simulink model "TorqueDistribution"  (R2024b)
settings: configuration reference "STM32H7_Config" (kept outside this file)
undefined symbols (not defined in the file): MMotorMaxAllowed, MMotorMinAllowed, MNominal, NKe
libraries: simulink x5
settings Model: DataDictionary=Master_Dictionary.sldd  EnableAccessToBaseWorkspace=off  Creator=torni  LastModifiedBy=William
settings ConfigSetRef: SourceName=STM32H7_Config

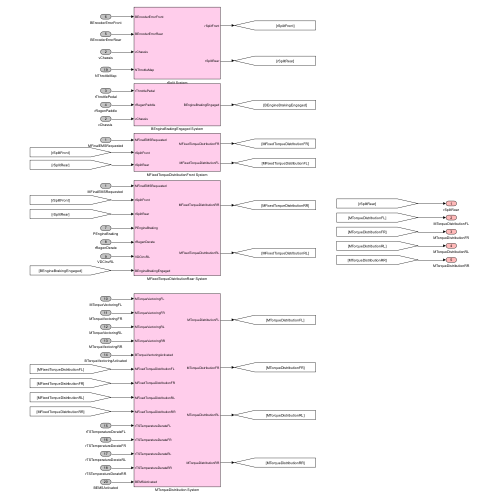
[thumbnail: Simulink's stored preview of the top-level diagram]
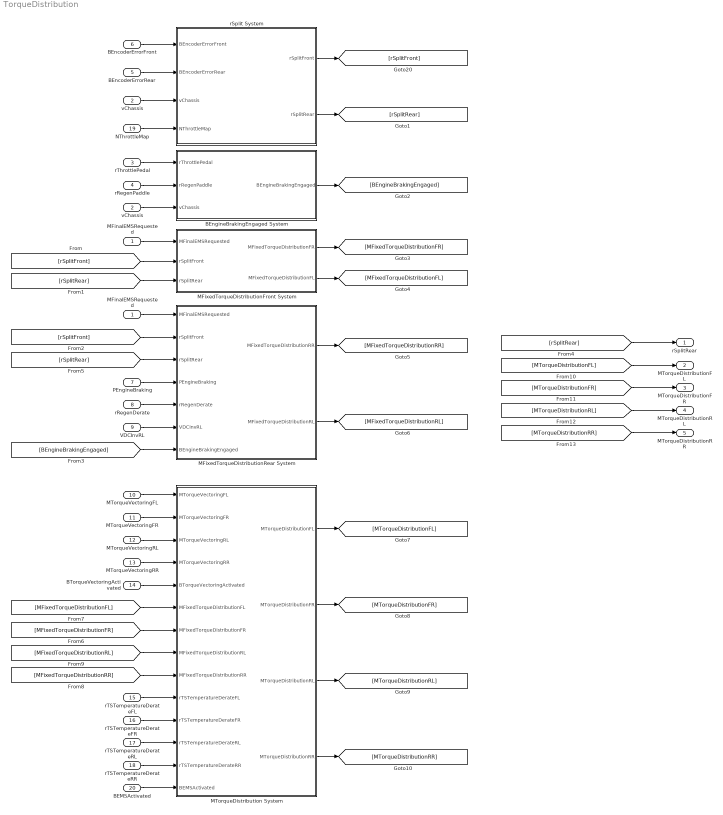
== system TorqueDistribution ==
  MFinalEMSRequested : Inport  OutDataTypeStr=double
  vChassis : Inport  Port=2  OutDataTypeStr=double
  "rThrottlePedal " : Inport  Port=3  OutDataTypeStr=double
  rRegenPaddle : Inport  Port=4  OutDataTypeStr=double
  BEncoderErrorRear : Inport  Port=5  OutDataTypeStr=boolean
  BEncoderErrorFront : Inport  Port=6  OutDataTypeStr=boolean
  PEngineBraking : Inport  Port=7  OutDataTypeStr=double
  rRegenDerate : Inport  Port=8  OutDataTypeStr=double
  VDCInvRL : Inport  Port=9  OutDataTypeStr=double
  MTorqueVectoringFL : Inport  Port=10  OutDataTypeStr=double
  MTorqueVectoringFR : Inport  Port=11  OutDataTypeStr=double
  MTorqueVectoringRL : Inport  Port=12  OutDataTypeStr=double
  MTorqueVectoringRR : Inport  Port=13  OutDataTypeStr=double
  BTorqueVectoringActivated : Inport  Port=14  OutDataTypeStr=boolean
  rTSTemperatureDerateFL : Inport  Port=15  OutDataTypeStr=double
  rTSTemperatureDerateFR : Inport  Port=16  OutDataTypeStr=double
  rTSTemperatureDerateRL : Inport  Port=17  OutDataTypeStr=double
  rTSTemperatureDerateRR : Inport  Port=18  OutDataTypeStr=double
  NThrottleMap : Inport  Port=19  OutDataTypeStr=double
  BEMSActivated : Inport  Port=20  OutDataTypeStr=boolean
  BEngineBrakingEngaged System : Subsystem
  "MFinalEMSRequested " : InportShadow  OutDataTypeStr=double
  MFixedTorqueDistributionFront System : Subsystem
  MFixedTorqueDistributionRear System : Subsystem
  MTorqueDistribution System : Subsystem
  rSplit System : Subsystem
  "vChassis " : InportShadow  Port=2  OutDataTypeStr=double
  rSplitRear : Outport  OutDataTypeStr=double  VectorParamsAs1DForOutWhenUnconnected=off
  MTorqueDistributionFL : Outport  Port=2  OutDataTypeStr=double  VectorParamsAs1DForOutWhenUnconnected=off
  MTorqueDistributionFR : Outport  Port=3  OutDataTypeStr=double  VectorParamsAs1DForOutWhenUnconnected=off
  MTorqueDistributionRL : Outport  Port=4  OutDataTypeStr=double  VectorParamsAs1DForOutWhenUnconnected=off
  MTorqueDistributionRR : Outport  Port=5  OutDataTypeStr=double  VectorParamsAs1DForOutWhenUnconnected=off
  wires:
  MFinalEMSRequested/1 -> MFixedTorqueDistributionFront System/1(MFinalEMSRequested)
  [rSplitRear] -> rSplitRear/1
  vChassis/1 -> rSplit System/3(vChassis)
  BEncoderErrorRear/1 -> rSplit System/2(BEncoderErrorRear)
  BEncoderErrorFront/1 -> rSplit System/1(BEncoderErrorFront)
  rSplit System/1(rSplitFront) -> [rSplitFront]
  rSplit System/2(rSplitRear) -> [rSplitRear]
  [rSplitFront] -> MFixedTorqueDistributionFront System/2(rSplitFront)
  [rSplitRear] -> MFixedTorqueDistributionFront System/3(rSplitRear)
  "rThrottlePedal "/1 -> BEngineBrakingEngaged System/1("rThrottlePedal ")
  rRegenPaddle/1 -> BEngineBrakingEngaged System/2(rRegenPaddle)
  BEngineBrakingEngaged System/1(BEngineBrakingEngaged) -> [BEngineBrakingEngaged]
  "MFinalEMSRequested "/1 -> MFixedTorqueDistributionRear System/1(MFinalEMSRequested)
  [rSplitFront] -> MFixedTorqueDistributionRear System/2(rSplitFront)
  [BEngineBrakingEngaged] -> MFixedTorqueDistributionRear System/7(BEngineBrakingEngaged)
  [rSplitRear] -> MFixedTorqueDistributionRear System/3(rSplitRear)
  PEngineBraking/1 -> MFixedTorqueDistributionRear System/4(PEngineBraking)
  rRegenDerate/1 -> MFixedTorqueDistributionRear System/5(rRegenDerate)
  VDCInvRL/1 -> MFixedTorqueDistributionRear System/6(VDCInvRL)
  MFixedTorqueDistributionFront System/1(MFixedTorqueDistributionFR) -> [MFixedTorqueDistributionFR]
  MFixedTorqueDistributionFront System/2(MFixedTorqueDistributionFL) -> [MFixedTorqueDistributionFL]
  MFixedTorqueDistributionRear System/1(MFixedTorqueDistributionRR) -> [MFixedTorqueDistributionRR]
  MFixedTorqueDistributionRear System/2(MFixedTorqueDistributionRL) -> [MFixedTorqueDistributionRL]
  [MFixedTorqueDistributionFL] -> MTorqueDistribution System/6("MFixedTorqueDistributionFL ")
  [MFixedTorqueDistributionFR] -> MTorqueDistribution System/7(MFixedTorqueDistributionFR)
  [MFixedTorqueDistributionRL] -> MTorqueDistribution System/8(MFixedTorqueDistributionRL)
  [MFixedTorqueDistributionRR] -> MTorqueDistribution System/9(MFixedTorqueDistributionRR)
  MTorqueVectoringFL/1 -> MTorqueDistribution System/1(MTorqueVectoringFL)
  MTorqueVectoringFR/1 -> MTorqueDistribution System/2(MTorqueVectoringFR)
  MTorqueVectoringRL/1 -> MTorqueDistribution System/3(MTorqueVectoringRL)
  MTorqueVectoringRR/1 -> MTorqueDistribution System/4(MTorqueVectoringRR)
  BTorqueVectoringActivated/1 -> MTorqueDistribution System/5(BTorqueVectoringActivated)
  MTorqueDistribution System/1(MTorqueDistributionFL) -> [MTorqueDistributionFL]
  MTorqueDistribution System/2(MTorqueDistributionFR) -> [MTorqueDistributionFR]
  MTorqueDistribution System/3(MTorqueDistributionRL) -> [MTorqueDistributionRL]
  MTorqueDistribution System/4(MTorqueDistributionRR) -> [MTorqueDistributionRR]
  [MTorqueDistributionFL] -> MTorqueDistributionFL/1
  [MTorqueDistributionFR] -> MTorqueDistributionFR/1
  [MTorqueDistributionRL] -> MTorqueDistributionRL/1
  [MTorqueDistributionRR] -> MTorqueDistributionRR/1
  rTSTemperatureDerateFL/1 -> MTorqueDistribution System/10(rTSTemperatureDerateFL)
  rTSTemperatureDerateFR/1 -> MTorqueDistribution System/11(rTSTemperatureDerateFR)
  rTSTemperatureDerateRL/1 -> MTorqueDistribution System/12(rTSTemperatureDerateRL)
  rTSTemperatureDerateRR/1 -> MTorqueDistribution System/13(rTSTemperatureDerateRR)
  "vChassis "/1 -> BEngineBrakingEngaged System/3(vChassis)
  NThrottleMap/1 -> rSplit System/4(NThrottleMap)
  BEMSActivated/1 -> MTorqueDistribution System/14(BEMSActivated)

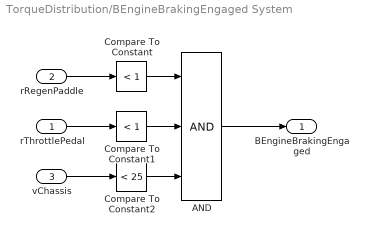
== system TorqueDistribution/BEngineBrakingEngaged System ==
  "rThrottlePedal " : Inport  OutDataTypeStr=double
  rRegenPaddle : Inport  Port=2  OutDataTypeStr=double
  vChassis : Inport  Port=3  OutDataTypeStr=double
  AND : Logic  Inputs=3  AllPortsSameDT=off  OutDataTypeStr=boolean
  Compare To Constant : simulink/Logic and Bit Operations/Compare To Constant  relop=<  const=1  OutDataTypeStr=boolean
  Compare To Constant1 : simulink/Logic and Bit Operations/Compare To Constant  relop=<  const=1  OutDataTypeStr=boolean
  Compare To Constant2 : simulink/Logic and Bit Operations/Compare To Constant  relop=<  const=25  OutDataTypeStr=boolean
  BEngineBrakingEngaged : Outport  OutDataTypeStr=boolean  VectorParamsAs1DForOutWhenUnconnected=off
  wires:
  AND/1 -> BEngineBrakingEngaged/1
  rRegenPaddle/1 -> Compare To Constant/1
  Compare To Constant1/1 -> AND/2
  Compare To Constant/1 -> AND/1
  "rThrottlePedal "/1 -> Compare To Constant1/1
  vChassis/1 -> Compare To Constant2/1
  Compare To Constant2/1 -> AND/3

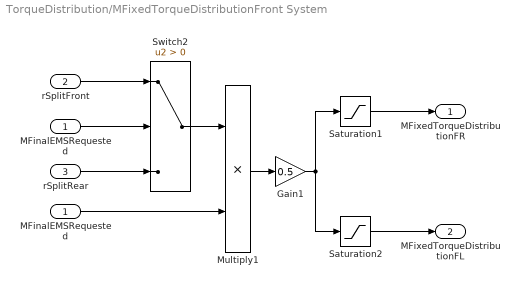
== system TorqueDistribution/MFixedTorqueDistributionFront System ==
  MFinalEMSRequested : Inport  OutDataTypeStr=double
  rSplitFront : Inport  Port=2  OutDataTypeStr=double
  rSplitRear : Inport  Port=3  OutDataTypeStr=double
  Gain1 : Gain  Gain=0.5
  "MFinalEMSRequested " : InportShadow  OutDataTypeStr=double
  Multiply1 : Product
  Saturation1 : Saturate  UpperLimit=MMotorMaxAllowed  LowerLimit=MMotorMinAllowed
  Saturation2 : Saturate  UpperLimit=MMotorMaxAllowed  LowerLimit=MMotorMinAllowed
  Switch2 : Switch  Criteria=u2 > Threshold  SaturateOnIntegerOverflow=off  InputSameDT=off
  MFixedTorqueDistributionFR : Outport  OutDataTypeStr=double  VectorParamsAs1DForOutWhenUnconnected=off
  MFixedTorqueDistributionFL : Outport  Port=2  OutDataTypeStr=double  VectorParamsAs1DForOutWhenUnconnected=off
  wires:
  Saturation2/1 -> MFixedTorqueDistributionFL/1
  Switch2/1 -> Multiply1/1
  Saturation1/1 -> MFixedTorqueDistributionFR/1
  Gain1/1 -> Saturation2/1, Saturation1/1
  Multiply1/1 -> Gain1/1
  MFinalEMSRequested/1 -> Switch2/2
  rSplitFront/1 -> Switch2/1
  rSplitRear/1 -> Switch2/3
  "MFinalEMSRequested "/1 -> Multiply1/2

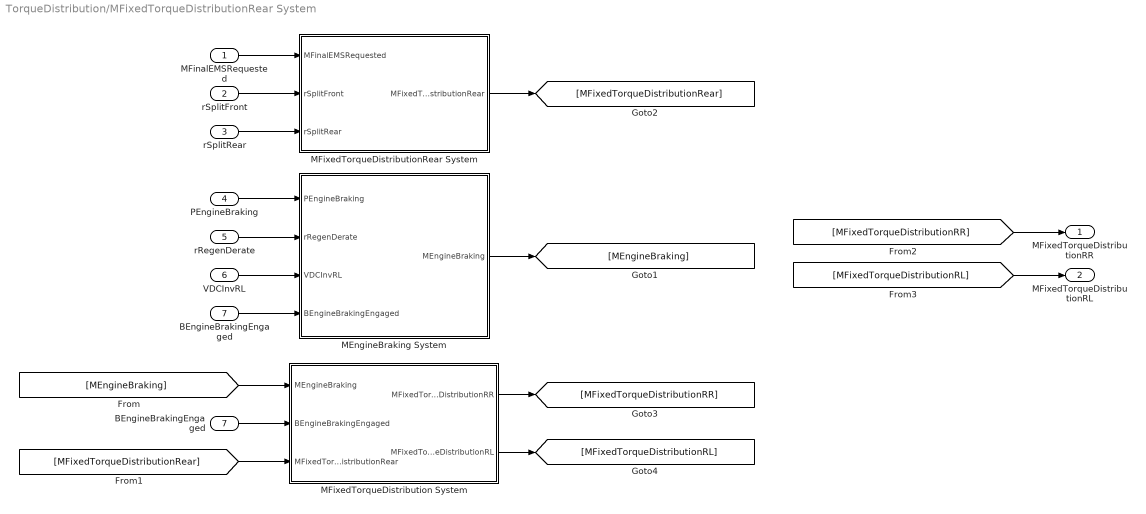
== system TorqueDistribution/MFixedTorqueDistributionRear System ==
  MFinalEMSRequested : Inport  OutDataTypeStr=double
  rSplitFront : Inport  Port=2  OutDataTypeStr=double
  rSplitRear : Inport  Port=3  OutDataTypeStr=double
  PEngineBraking : Inport  Port=4  OutDataTypeStr=double
  rRegenDerate : Inport  Port=5  OutDataTypeStr=double
  VDCInvRL : Inport  Port=6  OutDataTypeStr=double
  BEngineBrakingEngaged : Inport  Port=7  OutDataTypeStr=boolean
  "BEngineBrakingEngaged " : InportShadow  Port=7  OutDataTypeStr=boolean
  MEngineBraking System : Subsystem
  MFixedTorqueDistribution System : Subsystem
  MFixedTorqueDistributionRear System : Subsystem
  MFixedTorqueDistributionRR : Outport  OutDataTypeStr=double  VectorParamsAs1DForOutWhenUnconnected=off
  MFixedTorqueDistributionRL : Outport  Port=2  OutDataTypeStr=double  VectorParamsAs1DForOutWhenUnconnected=off
  wires:
  MFinalEMSRequested/1 -> MFixedTorqueDistributionRear System/1(MFinalEMSRequested)
  rSplitFront/1 -> MFixedTorqueDistributionRear System/2(rSplitFront)
  rSplitRear/1 -> MFixedTorqueDistributionRear System/3(rSplitRear)
  MFixedTorqueDistributionRear System/1(MFixedTorqueDistributionRear) -> [MFixedTorqueDistributionRear]
  PEngineBraking/1 -> MEngineBraking System/1(PEngineBraking)
  rRegenDerate/1 -> MEngineBraking System/2(rRegenDerate)
  VDCInvRL/1 -> MEngineBraking System/3(VDCInvRL)
  BEngineBrakingEngaged/1 -> MEngineBraking System/4(BEngineBrakingEngaged)
  MEngineBraking System/1(MEngineBraking) -> [MEngineBraking]
  "BEngineBrakingEngaged "/1 -> MFixedTorqueDistribution System/2(BEngineBrakingEngaged)
  [MEngineBraking] -> MFixedTorqueDistribution System/1(MEngineBraking)
  [MFixedTorqueDistributionRear] -> MFixedTorqueDistribution System/3(MFixedTorqueDistributionRear)
  MFixedTorqueDistribution System/1(MFixedTorqueDistributionRR) -> [MFixedTorqueDistributionRR]
  MFixedTorqueDistribution System/2(MFixedTorqueDistributionRL) -> [MFixedTorqueDistributionRL]
  [MFixedTorqueDistributionRR] -> MFixedTorqueDistributionRR/1
  [MFixedTorqueDistributionRL] -> MFixedTorqueDistributionRL/1

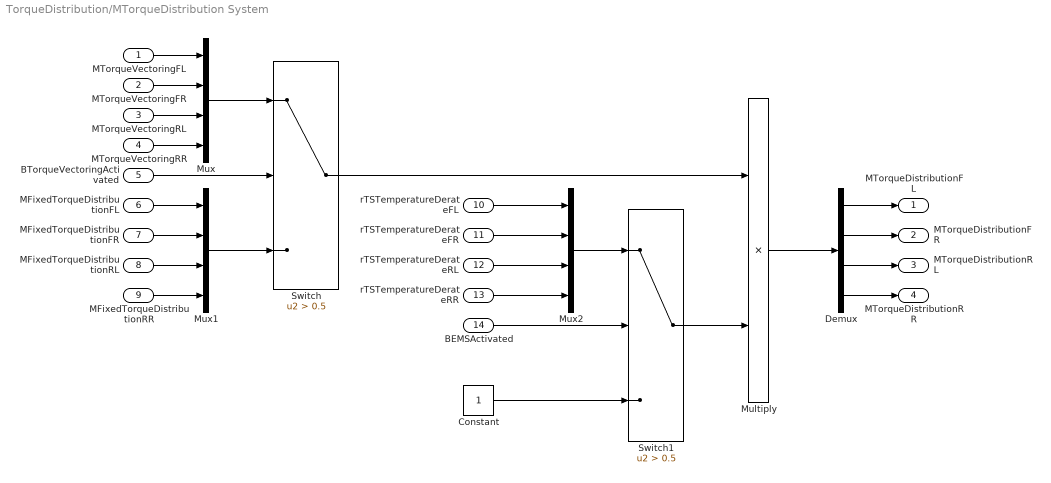
== system TorqueDistribution/MTorqueDistribution System ==
  MTorqueVectoringFL : Inport  OutDataTypeStr=double
  MTorqueVectoringFR : Inport  Port=2  OutDataTypeStr=double
  MTorqueVectoringRL : Inport  Port=3  OutDataTypeStr=double
  MTorqueVectoringRR : Inport  Port=4  OutDataTypeStr=double
  BTorqueVectoringActivated : Inport  Port=5  OutDataTypeStr=boolean
  "MFixedTorqueDistributionFL " : Inport  Port=6  OutDataTypeStr=double
  MFixedTorqueDistributionFR : Inport  Port=7  OutDataTypeStr=double
  MFixedTorqueDistributionRL : Inport  Port=8  OutDataTypeStr=double
  MFixedTorqueDistributionRR : Inport  Port=9  OutDataTypeStr=double
  rTSTemperatureDerateFL : Inport  Port=10  OutDataTypeStr=double
  rTSTemperatureDerateFR : Inport  Port=11  OutDataTypeStr=double
  rTSTemperatureDerateRL : Inport  Port=12  OutDataTypeStr=double
  rTSTemperatureDerateRR : Inport  Port=13  OutDataTypeStr=double
  BEMSActivated : Inport  Port=14  OutDataTypeStr=boolean
  Constant : Constant
  Demux : Demux
  Multiply : Product
  Mux : Mux
  Mux1 : Mux
  Mux2 : Mux
  Switch : Switch  Criteria=u2 > Threshold  Threshold=0.5  SaturateOnIntegerOverflow=off  InputSameDT=off
  Switch1 : Switch  Criteria=u2 > Threshold  Threshold=0.5  SaturateOnIntegerOverflow=off  InputSameDT=off
  MTorqueDistributionFL : Outport  OutDataTypeStr=double  VectorParamsAs1DForOutWhenUnconnected=off
  MTorqueDistributionFR : Outport  Port=2  OutDataTypeStr=double  VectorParamsAs1DForOutWhenUnconnected=off
  MTorqueDistributionRL : Outport  Port=3  OutDataTypeStr=double  VectorParamsAs1DForOutWhenUnconnected=off
  MTorqueDistributionRR : Outport  Port=4  OutDataTypeStr=double  VectorParamsAs1DForOutWhenUnconnected=off
  wires:
  BTorqueVectoringActivated/1 -> Switch/2
  rTSTemperatureDerateFL/1 -> Mux2/1
  Demux/2 -> MTorqueDistributionFR/1
  Demux/3 -> MTorqueDistributionRL/1
  Mux2/1 -> Switch1/1
  MFixedTorqueDistributionRR/1 -> Mux1/4
  Constant/1 -> Switch1/3
  Switch1/1 -> Multiply/2
  MTorqueVectoringRR/1 -> Mux/4
  MTorqueVectoringFR/1 -> Mux/2
  MTorqueVectoringFL/1 -> Mux/1
  MTorqueVectoringRL/1 -> Mux/3
  Switch/1 -> Multiply/1
  rTSTemperatureDerateFR/1 -> Mux2/2
  "MFixedTorqueDistributionFL "/1 -> Mux1/1
  Demux/4 -> MTorqueDistributionRR/1
  rTSTemperatureDerateRR/1 -> Mux2/4
  Mux1/1 -> Switch/3
  MFixedTorqueDistributionFR/1 -> Mux1/2
  rTSTemperatureDerateRL/1 -> Mux2/3
  Demux/1 -> MTorqueDistributionFL/1
  BEMSActivated/1 -> Switch1/2
  Mux/1 -> Switch/1
  MFixedTorqueDistributionRL/1 -> Mux1/3
  Multiply/1 -> Demux/1

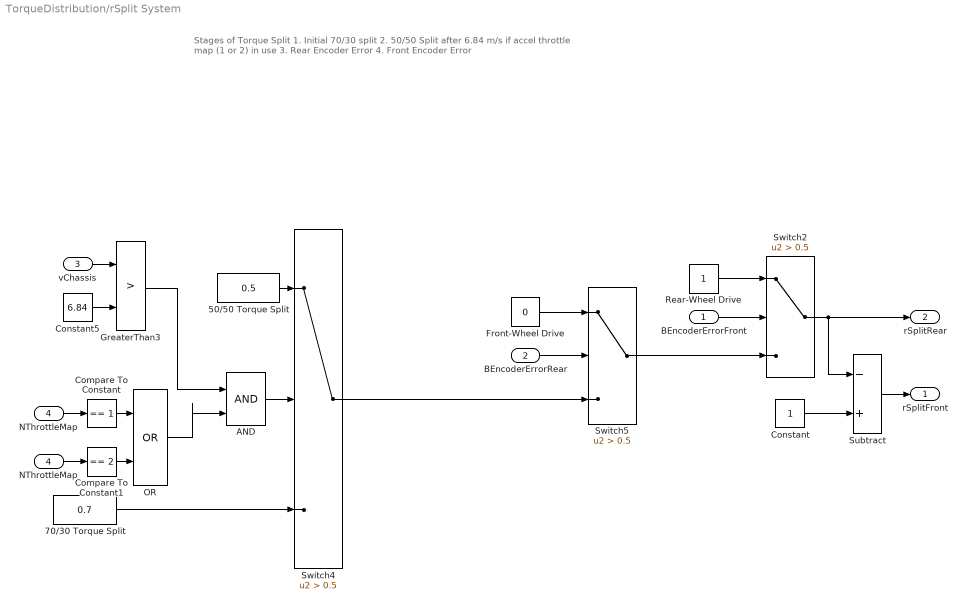
== system TorqueDistribution/rSplit System ==
  note: Stages of Torque Split
      | 1. Initial 70/30 split
      | 2. 50/50 Split after 6.84 m/s if accel throttle map (1 or 2) in use
      | 3. Rear Encoder Error
      | 4. Front Encoder Error
  BEncoderErrorFront : Inport  OutDataTypeStr=boolean
  BEncoderErrorRear : Inport  Port=2  OutDataTypeStr=boolean
  vChassis : Inport  Port=3  OutDataTypeStr=double
  NThrottleMap : Inport  Port=4  OutDataTypeStr=double
  50/50 Torque Split : Constant  Value=0.5
  70/30 Torque Split : Constant  Value=0.7
  AND : Logic  IconShape=distinctive  AllPortsSameDT=off  OutDataTypeStr=boolean
  Compare To Constant : simulink/Logic and Bit Operations/Compare To Constant  relop===  const=1  OutDataTypeStr=boolean
  Compare To Constant1 : simulink/Logic and Bit Operations/Compare To Constant  relop===  const=2  OutDataTypeStr=boolean
  Constant : Constant
  Constant5 : Constant  Value=6.84
  Front-Wheel Drive : Constant  Value=0
  GreaterThan3 : RelationalOperator  Operator=>  OutDataTypeStr=boolean  RndMeth=Simplest  InputSameDT=off
  "NThrottleMap " : InportShadow  Port=4  OutDataTypeStr=double
  OR : Logic  Operator=OR  IconShape=distinctive  AllPortsSameDT=off  OutDataTypeStr=boolean
  Rear-Wheel Drive : Constant
  Subtract : Sum  Inputs=-+
  Switch2 : Switch  Criteria=u2 > Threshold  Threshold=0.5  SaturateOnIntegerOverflow=off  InputSameDT=off
  Switch4 : Switch  Criteria=u2 > Threshold  Threshold=0.5  SaturateOnIntegerOverflow=off  InputSameDT=off
  Switch5 : Switch  Criteria=u2 > Threshold  Threshold=0.5  SaturateOnIntegerOverflow=off  InputSameDT=off
  rSplitFront : Outport  OutDataTypeStr=double  VectorParamsAs1DForOutWhenUnconnected=off
  rSplitRear : Outport  Port=2  OutDataTypeStr=double  VectorParamsAs1DForOutWhenUnconnected=off
  wires:
  BEncoderErrorFront/1 -> Switch2/2
  Rear-Wheel Drive/1 -> Switch2/1
  Switch2/1 -> rSplitRear/1, Subtract/1
  Switch5/1 -> Switch2/3
  Front-Wheel Drive/1 -> Switch5/1
  BEncoderErrorRear/1 -> Switch5/2
  Subtract/1 -> rSplitFront/1
  Constant/1 -> Subtract/2
  50/50 Torque Split/1 -> Switch4/1
  vChassis/1 -> GreaterThan3/1
  Switch4/1 -> Switch5/3
  AND/1 -> Switch4/2
  Constant5/1 -> GreaterThan3/2
  GreaterThan3/1 -> AND/1
  OR/1 -> AND/2
  Compare To Constant/1 -> OR/1
  NThrottleMap/1 -> Compare To Constant/1
  Compare To Constant1/1 -> OR/2
  "NThrottleMap "/1 -> Compare To Constant1/1
  70/30 Torque Split/1 -> Switch4/3

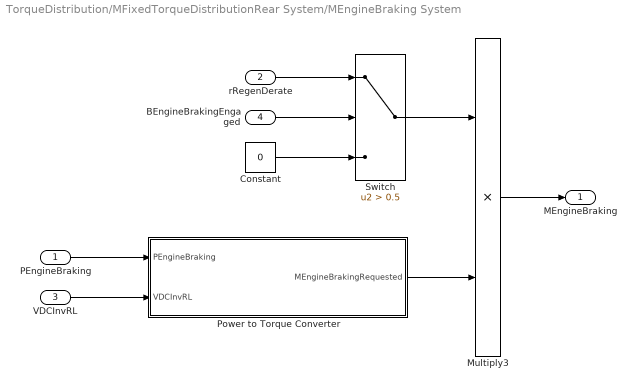
== system TorqueDistribution/MFixedTorqueDistributionRear System/MEngineBraking System ==
  PEngineBraking : Inport  OutDataTypeStr=double
  rRegenDerate : Inport  Port=2  OutDataTypeStr=double
  VDCInvRL : Inport  Port=3  OutDataTypeStr=double
  BEngineBrakingEngaged : Inport  Port=4  OutDataTypeStr=boolean
  Constant : Constant  Value=0
  Multiply3 : Product
  Power to Torque Converter : Subsystem
  Switch : Switch  Criteria=u2 > Threshold  Threshold=0.5  SaturateOnIntegerOverflow=off  InputSameDT=off
  MEngineBraking : Outport  OutDataTypeStr=double  VectorParamsAs1DForOutWhenUnconnected=off
  wires:
  VDCInvRL/1 -> Power to Torque Converter/2(VDCInvRL)
  Power to Torque Converter/1(MEngineBrakingRequested) -> Multiply3/2
  rRegenDerate/1 -> Switch/1
  Multiply3/1 -> MEngineBraking/1
  Switch/1 -> Multiply3/1
  PEngineBraking/1 -> Power to Torque Converter/1(PEngineBraking)
  BEngineBrakingEngaged/1 -> Switch/2
  Constant/1 -> Switch/3

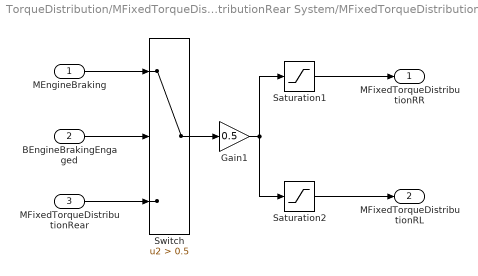
== system TorqueDistribution/MFixedTorqueDistributionRear System/MFixedTorqueDistribution System ==
  MEngineBraking : Inport  OutDataTypeStr=double
  BEngineBrakingEngaged : Inport  Port=2  OutDataTypeStr=boolean
  MFixedTorqueDistributionRear : Inport  Port=3  OutDataTypeStr=double
  Gain1 : Gain  Gain=0.5
  Saturation1 : Saturate  UpperLimit=MMotorMaxAllowed  LowerLimit=MMotorMinAllowed
  Saturation2 : Saturate  UpperLimit=MMotorMaxAllowed  LowerLimit=MMotorMinAllowed
  Switch : Switch  Criteria=u2 > Threshold  Threshold=0.5  SaturateOnIntegerOverflow=off  InputSameDT=off
  MFixedTorqueDistributionRR : Outport  OutDataTypeStr=double  VectorParamsAs1DForOutWhenUnconnected=off
  MFixedTorqueDistributionRL : Outport  Port=2  OutDataTypeStr=double  VectorParamsAs1DForOutWhenUnconnected=off
  wires:
  BEngineBrakingEngaged/1 -> Switch/2
  Saturation1/1 -> MFixedTorqueDistributionRR/1
  Saturation2/1 -> MFixedTorqueDistributionRL/1
  Gain1/1 -> Saturation1/1, Saturation2/1
  Switch/1 -> Gain1/1
  MFixedTorqueDistributionRear/1 -> Switch/3
  MEngineBraking/1 -> Switch/1

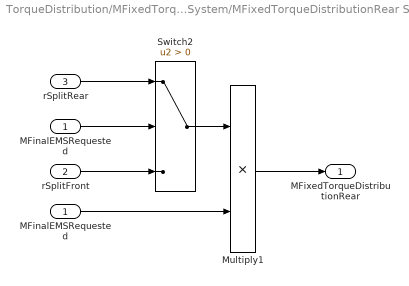
== system TorqueDistribution/MFixedTorqueDistributionRear System/MFixedTorqueDistributionRear System ==
  MFinalEMSRequested : Inport  OutDataTypeStr=double
  rSplitFront : Inport  Port=2  OutDataTypeStr=double
  rSplitRear : Inport  Port=3  OutDataTypeStr=double
  "MFinalEMSRequested " : InportShadow  OutDataTypeStr=double
  Multiply1 : Product
  Switch2 : Switch  Criteria=u2 > Threshold  SaturateOnIntegerOverflow=off  InputSameDT=off
  MFixedTorqueDistributionRear : Outport  OutDataTypeStr=double  VectorParamsAs1DForOutWhenUnconnected=off
  wires:
  rSplitFront/1 -> Switch2/3
  MFinalEMSRequested/1 -> Switch2/2
  "MFinalEMSRequested "/1 -> Multiply1/2
  Switch2/1 -> Multiply1/1
  rSplitRear/1 -> Switch2/1
  Multiply1/1 -> MFixedTorqueDistributionRear/1

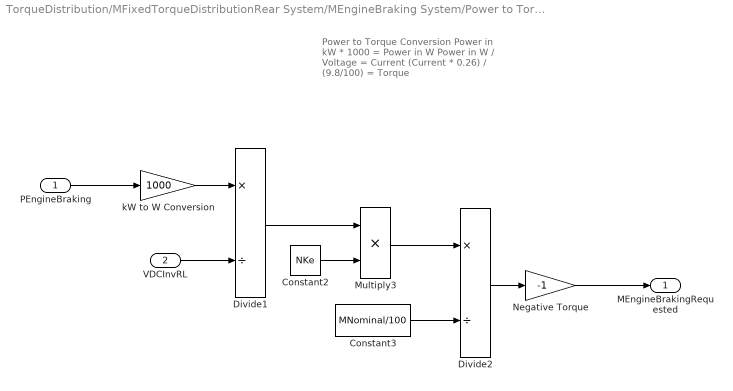
== system TorqueDistribution/MFixedTorqueDistributionRear System/MEngineBraking System/Power to Torque Converter ==
  note: Power to Torque Conversion
      |
      | Power in kW * 1000 = Power in W
      |
      | Power in W / Voltage = Current
      |
      | (Current * 0.26) / (9.8/100) = Torque
  PEngineBraking : Inport  OutDataTypeStr=double
  VDCInvRL : Inport  Port=2  OutDataTypeStr=double
  Constant2 : Constant  Value=NKe
  Constant3 : Constant  Value=MNominal/100
  Divide1 : Product  Inputs=*/
  Divide2 : Product  Inputs=*/
  Multiply3 : Product
  Negative Torque : Gain  Gain=-1
  kW to W Conversion : Gain  Gain=1000
  MEngineBrakingRequested : Outport  OutDataTypeStr=double  VectorParamsAs1DForOutWhenUnconnected=off
  wires:
  VDCInvRL/1 -> Divide1/2
  kW to W Conversion/1 -> Divide1/1
  Multiply3/1 -> Divide2/1
  PEngineBraking/1 -> kW to W Conversion/1
  Constant2/1 -> Multiply3/2
  Divide2/1 -> Negative Torque/1
  Divide1/1 -> Multiply3/1
  Constant3/1 -> Divide2/2
  Negative Torque/1 -> MEngineBrakingRequested/1
